simulink subsystem "rss_RefTqLimCalc"  (R2023a)
settings: Solver=VariableStepAuto  StartTime=0.0  StopTime=inf  RelTol=1e-3
undefined symbols (not defined in the file): bit, Cdbl_iPhCurrMaxVal, Cdbl_iPhCurrPeakVal, Cdbl_iSplyCurrMaxVal, Cdbl_numPPNumMaxVal, Cdbl_psiPermMagFlxMaxVal, Cdbl_psiPermMagFlxMinVal, Cdbl_psiPermMagFlxPeakVal, Cdbl_trqTqMaxVal, Cdbl_trqTqPeakVal, Cdbl_uPhVltgMaxVal, Cdbl_uSplyVltgMaxVal, Gs16_iPhCurrLim_CUR, Gs16_iPhCurrLim_CUR_tPCBTemp_X, Gs16_iSplyCurrTempLim_CUR, Gs16_iSplyCurrTempLim_CUR_tPCBTemp_X, Gs16_iSplyCurrVltgLim_CUR, Gs16_iSplyCurrVltgLim_CUR_uSplyVltg_X
libraries: lib_conversion x9, lib_configurable_parameter x3, lib_dynamic_saturator x2, simulink x1, lib_iir_filter x1
settings Model: DefaultTestHarness=rss_DeratingControl_thu  Creator=CAV2OFO  LastModifiedBy=xiaoqiang.yuan
settings OptimizationCC: ReuseModelBlockBuffer=off

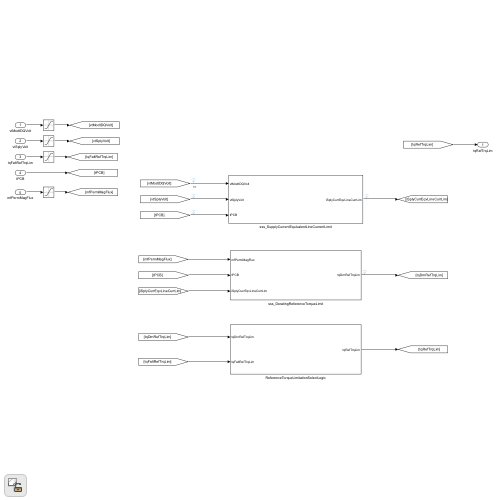
[thumbnail: Simulink's stored preview of the top-level diagram]
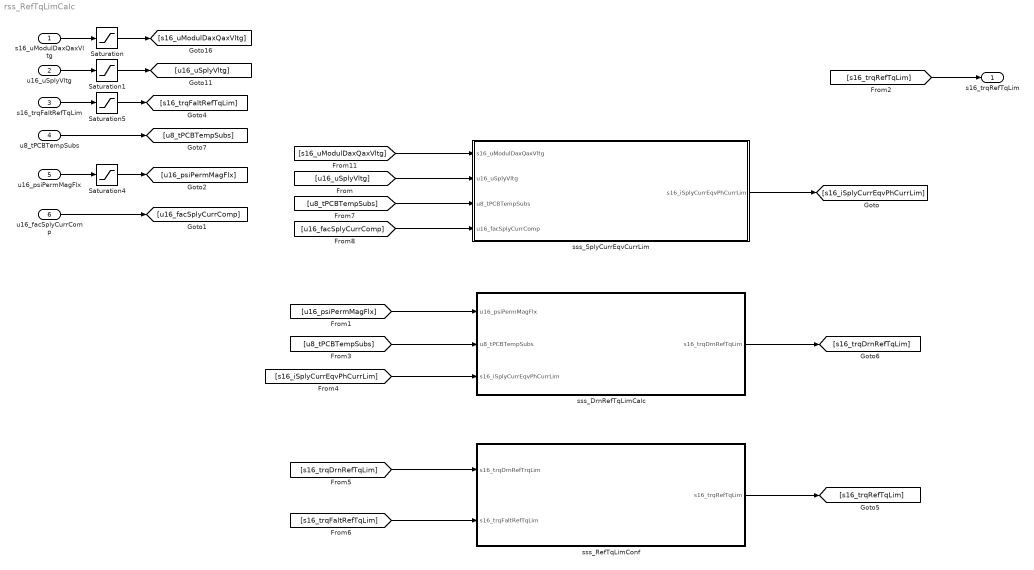
== system rss_RefTqLimCalc ==
  s16_uModulDaxQaxVltg : Inport  OutDataTypeStr=dt_Standardize_s16p15b0
  u16_uSplyVltg : Inport  Port=2  OutDataTypeStr=dt_Standardize_u16p15b0
  s16_trqFaltRefTqLim : Inport  Port=3  OutDataTypeStr=dt_Standardize_s16p15b0
  u8_tPCBTempSubs : Inport  Port=4  OutDataTypeStr=dt_Temp_u8p0bn40
  u16_psiPermMagFlx : Inport  Port=5  OutDataTypeStr=dt_Standardize_u16p15b0
  u16_facSplyCurrComp : Inport  Port=6  OutDataTypeStr=dt_Standardize_u16p15b0
  Saturation : Saturate  UpperLimit=Cdbl_uPhVltgMaxVal  LowerLimit=-Cdbl_uPhVltgMaxVal
  Saturation1 : Saturate  UpperLimit=Cdbl_uSplyVltgMaxVal  LowerLimit=0
  Saturation4 : Saturate  UpperLimit=Cdbl_psiPermMagFlxMaxVal  LowerLimit=Cdbl_psiPermMagFlxMinVal
  Saturation5 : Saturate  UpperLimit=Cdbl_trqTqMaxVal  LowerLimit=-Cdbl_trqTqMaxVal  LinearizeAsGain=off
  sss_DrnRefTqLimCalc : Subsystem
  sss_RefTqLimConf : Subsystem
  sss_SplyCurrEqvCurrLim : Subsystem
  s16_trqRefTqLim : Outport  OutDataTypeStr=dt_Standardize_s16p15b0
  wires:
  [s16_trqRefTqLim] -> s16_trqRefTqLim/1
  s16_uModulDaxQaxVltg/1 -> Saturation/1
  u16_uSplyVltg/1 -> Saturation1/1
  [u16_uSplyVltg] -> sss_SplyCurrEqvCurrLim/2(u16_uSplyVltg)
  [s16_uModulDaxQaxVltg] -> sss_SplyCurrEqvCurrLim/1(s16_uModulDaxQaxVltg)
  sss_SplyCurrEqvCurrLim/1(s16_iSplyCurrEqvPhCurrLim) -> [s16_iSplyCurrEqvPhCurrLim]
  [u16_psiPermMagFlx] -> sss_DrnRefTqLimCalc/1(u16_psiPermMagFlx)
  [u8_tPCBTempSubs] -> sss_DrnRefTqLimCalc/2(u8_tPCBTempSubs)
  [s16_iSplyCurrEqvPhCurrLim] -> sss_DrnRefTqLimCalc/3(s16_iSplyCurrEqvPhCurrLim)
  Saturation/1 -> [s16_uModulDaxQaxVltg]
  Saturation1/1 -> [u16_uSplyVltg]
  Saturation4/1 -> [u16_psiPermMagFlx]
  s16_trqFaltRefTqLim/1 -> Saturation5/1
  Saturation5/1 -> [s16_trqFaltRefTqLim]
  sss_RefTqLimConf/1(s16_trqRefTqLim) -> [s16_trqRefTqLim]
  sss_DrnRefTqLimCalc/1(s16_trqDrnRefTqLim) -> [s16_trqDrnRefTqLim]
  [s16_trqDrnRefTqLim] -> sss_RefTqLimConf/1(s16_trqDrnRefTrqLim)
  [s16_trqFaltRefTqLim] -> sss_RefTqLimConf/2(s16_trqFaltRefTqLim)
  u8_tPCBTempSubs/1 -> [u8_tPCBTempSubs]
  [u8_tPCBTempSubs] -> sss_SplyCurrEqvCurrLim/3(u8_tPCBTempSubs)
  u16_psiPermMagFlx/1 -> Saturation4/1
  u16_facSplyCurrComp/1 -> [u16_facSplyCurrComp]
  [u16_facSplyCurrComp] -> sss_SplyCurrEqvCurrLim/4(u16_facSplyCurrComp)

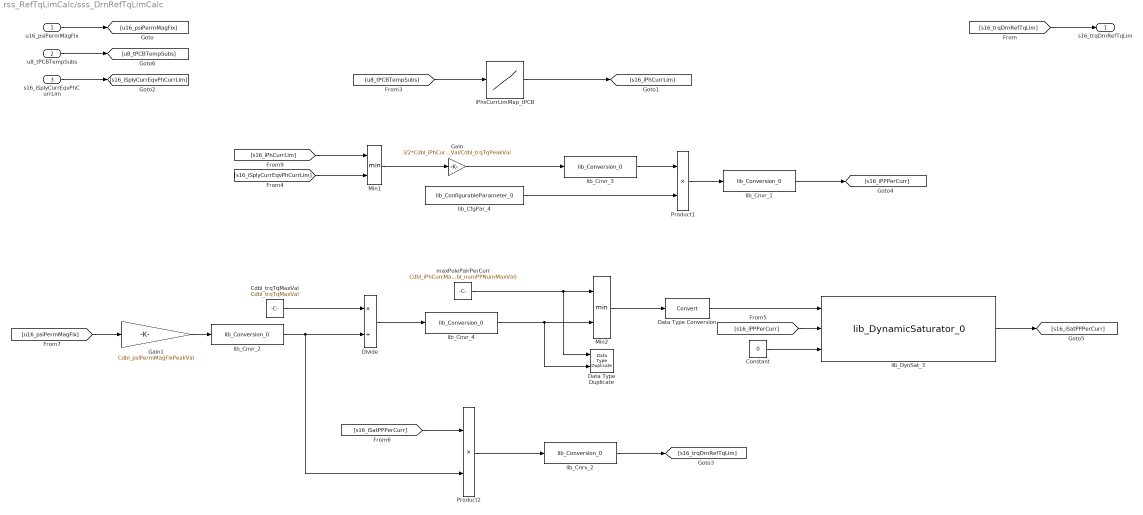
== system rss_RefTqLimCalc/sss_DrnRefTqLimCalc ==
  u16_psiPermMagFlx : Inport
  u8_tPCBTempSubs : Inport  Port=2
  s16_iSplyCurrEqvPhCurrLim : Inport  Port=3
  Cdbl_trqTqMaxVal : Constant  Value=Cdbl_trqTqMaxVal  OutDataTypeStr=dt_Standardize_s16p15b0
  Constant : Constant  Value=0  OutDataTypeStr=Inherit: Inherit via back propagation
  Data Type Duplicate : DataTypeDuplicate
  Data Type Conversion : DataTypeConversion  SaturateOnIntegerOverflow=off  RndMeth=Floor
  Divide : Product  Inputs=*/  OutDataTypeStr=Inherit: Inherit via back propagation  RndMeth=Simplest
  Gain : Gain  Gain=3/2*Cdbl_iPhCurrPeakVal/Cdbl_trqTqPeakVal  OutDataTypeStr=Inherit: Inherit via back propagation
  Gain1 : Gain  Gain=Cdbl_psiPermMagFlxPeakVal  OutDataTypeStr=Inherit: Inherit via back propagation
  Min1 : MinMax  Inputs=2
  Min2 : MinMax  Inputs=2
  Product1 : Product  OutDataTypeStr=Inherit: Inherit via back propagation
  Product2 : Product  OutDataTypeStr=dt_Standardize_s16p15b0
  iPhsCurrLimMap_tPCB : Lookup_n-D  NumberOfTableDimensions=1  BreakpointsForDimension1=Gs16_iPhCurrLim_CUR_tPCBTemp_X  Table=Gs16_iPhCurrLim_CUR  ExtrapMethod=Clip  InternalRulePriority=Speed  OutDataTypeStr=Inherit: Inherit from 'Table data'  RndMeth=Simplest
  lib_CfgPar_4 : lib_configurable_parameter/lib_ConfigurableParameter_0  lb_parCnfgPar=Gu8_numPPNum_C  lb_parDataType=Inherit: Inherit from 'Constant value'  lb_parUpLim=Cdbl_numPPNumMaxVal  lb_parLowLim=Cdbl_numPPNumMinVal
  lib_Cnrv_2 : lib_conversion/lib_Conversion_0  lb_parDataType=dt_Standardize_s16p15b0  lb_parOutpMaxVal=[]  lb_parOutpMinVal=[]  RndMeth=Simplest  lb_parSatFlag=off
  lib_Cnvr_1 : lib_conversion/lib_Conversion_0  lb_parDataType=fixdt(0,16)  lb_parOutpMaxVal=Cdbl_iPhCurrMaxVal*3/2*Cdbl_iPhCurrPeakVal/Cdbl_trqTqPeakVal*double(Cdbl_numPPNumMaxVal)  lb_parOutpMinVal=[]  RndMeth=Simplest  lb_parSatFlag=off
  lib_Cnvr_2 : lib_conversion/lib_Conversion_0  lb_parDataType=fixdt(0,16)  lb_parOutpMaxVal=Cdbl_psiPermMagFlxPeakVal  lb_parOutpMinVal=[]  RndMeth=Simplest  lb_parSatFlag=off
  lib_Cnvr_3 : lib_conversion/lib_Conversion_0  lb_parDataType=fixdt(0,16)  lb_parOutpMaxVal=Cdbl_iPhCurrMaxVal*3/2*Cdbl_iPhCurrPeakVal/Cdbl_trqTqPeakVal  lb_parOutpMinVal=[]  RndMeth=Simplest  lb_parSatFlag=off
  lib_Cnvr_4 : lib_conversion/lib_Conversion_0  lb_parDataType=fixdt(0,16)  lb_parOutpMaxVal=Cdbl_trqTqMaxVal/Cdbl_psiPermMagFlxMinVal  lb_parOutpMinVal=[]  RndMeth=Simplest  lb_parSatFlag=off
  lib_DynSat_3 : lib_dynamic_saturator/lib_DynamicSaturator_0
  maxPolePairPerCurr : Constant  Value=Cdbl_iPhCurrMaxVal*3/2*Cdbl_iPhCurrPeakVal/Cdbl_trqTqPeakVal*double(Cdbl_numPPNumMaxVal)  OutDataTypeStr=Inherit: Inherit via back propagation
  s16_trqDrnRefTqLim : Outport
  wires:
  [u16_psiPermMagFlx] -> Gain1/1
  Gain1/1 -> lib_Cnvr_2/1
  iPhsCurrLimMap_tPCB/1 -> [s16_iPhCurrLim]
  [u8_tPCBTempSubs] -> iPhsCurrLimMap_tPCB/1
  u8_tPCBTempSubs/1 -> [u8_tPCBTempSubs]
  lib_Cnrv_2/1 -> [s16_trqDrnRefTqLim]
  Min2/1 -> Data Type Conversion/1
  maxPolePairPerCurr/1 -> Min2/1, Data Type Duplicate/1
  Data Type Conversion/1 -> lib_DynSat_3/1
  lib_Cnvr_4/1 -> Min2/2, Data Type Duplicate/2
  lib_Cnvr_3/1 -> Product1/1
  [s16_iSatPPPerCurr] -> Product2/1
  lib_DynSat_3/1 -> [s16_iSatPPPerCurr]
  [s16_iPPPerCurr] -> lib_DynSat_3/2
  Divide/1 -> lib_Cnvr_4/1
  lib_Cnvr_1/1 -> [s16_iPPPerCurr]
  Cdbl_trqTqMaxVal/1 -> Divide/1
  Constant/1 -> lib_DynSat_3/3
  [s16_trqDrnRefTqLim] -> s16_trqDrnRefTqLim/1
  s16_iSplyCurrEqvPhCurrLim/1 -> [s16_iSplyCurrEqvPhCurrLim]
  [s16_iSplyCurrEqvPhCurrLim] -> Min1/2
  [s16_iPhCurrLim] -> Min1/1
  u16_psiPermMagFlx/1 -> [u16_psiPermMagFlx]
  Product2/1 -> lib_Cnrv_2/1
  Product1/1 -> lib_Cnvr_1/1
  Gain/1 -> lib_Cnvr_3/1
  lib_CfgPar_4/1 -> Product1/2
  Min1/1 -> Gain/1
  lib_Cnvr_2/1 -> Product2/2, Divide/2

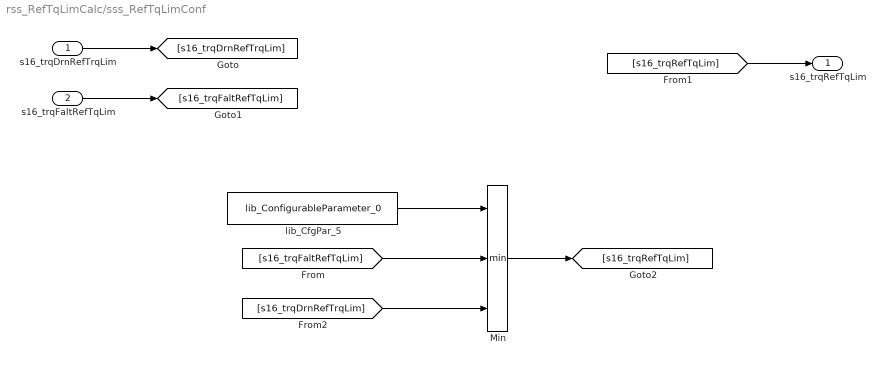
== system rss_RefTqLimCalc/sss_RefTqLimConf ==
  s16_trqDrnRefTrqLim : Inport
  s16_trqFaltRefTqLim : Inport  Port=2
  Min : MinMax  Inputs=3
  lib_CfgPar_5 : lib_configurable_parameter/lib_ConfigurableParameter_0  lb_parCnfgPar=Gs16_trqTqUpLim_C  lb_parDataType=Inherit: Inherit from 'Constant value'  lb_parUpLim=Cdbl_trqTqMaxVal  lb_parLowLim=0
  s16_trqRefTqLim : Outport
  wires:
  Min/1 -> [s16_trqRefTqLim]
  [s16_trqRefTqLim] -> s16_trqRefTqLim/1
  [s16_trqDrnRefTrqLim] -> Min/3
  s16_trqFaltRefTqLim/1 -> [s16_trqFaltRefTqLim]
  [s16_trqFaltRefTqLim] -> Min/2
  s16_trqDrnRefTrqLim/1 -> [s16_trqDrnRefTrqLim]
  lib_CfgPar_5/1 -> Min/1

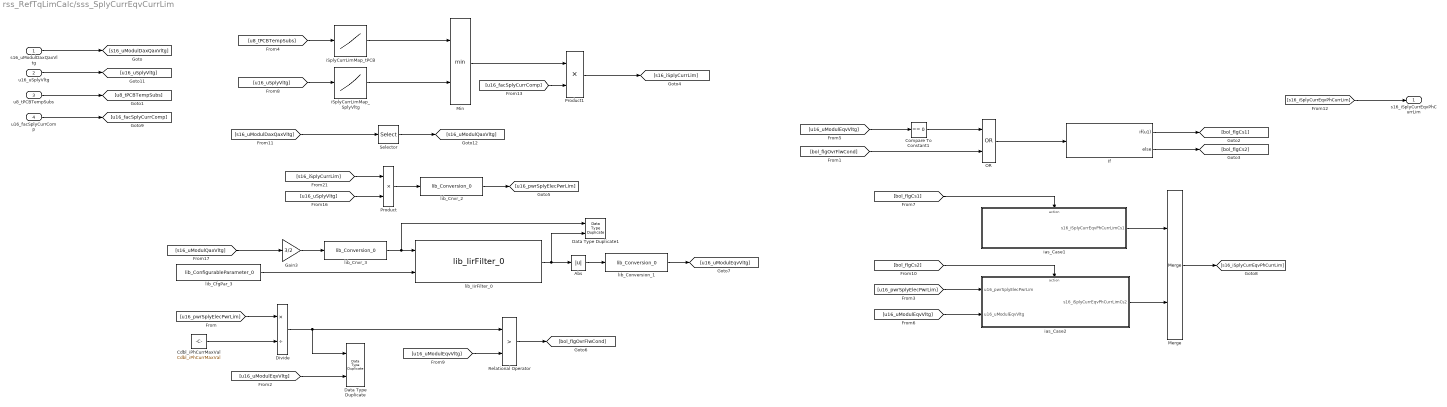
== system rss_RefTqLimCalc/sss_SplyCurrEqvCurrLim ==
  s16_uModulDaxQaxVltg : Inport
  u16_uSplyVltg : Inport  Port=2
  u8_tPCBTempSubs : Inport  Port=3
  u16_facSplyCurrComp : Inport  Port=4
  Abs : Abs  OutDataTypeStr=Inherit: Inherit via back propagation  RndMeth=Simplest  SaturateOnIntegerOverflow=off
  Cdbl_iPhCurrMaxVal : Constant  Value=Cdbl_iPhCurrMaxVal  OutDataTypeStr=dt_Standardize_s16p15b0
  Compare To Constant1 : simulink/Logic and Bit Operations/Compare To Constant  relop===  const=0  OutDataTypeStr=boolean
  Data Type Duplicate : DataTypeDuplicate
  Data Type Duplicate1 : DataTypeDuplicate
  Divide : Product  Inputs=*/  OutDataTypeStr=Inherit: Inherit via back propagation  RndMeth=Simplest
  Gain3 : Gain  Gain=3/2  OutDataTypeStr=Inherit: Inherit via back propagation  RndMeth=Simplest
  If : If  IfExpression=u1
  Merge : Merge
  Min : MinMax  Inputs=2
  OR : Logic  Operator=OR  AllPortsSameDT=off  OutDataTypeStr=boolean
  Product : Product  OutDataTypeStr=Inherit: Inherit via back propagation  RndMeth=Simplest
  Product1 : Product  RndMeth=Simplest  OutDataTypeStr=Inherit: Same as first input
  Relational Operator : RelationalOperator  Operator=>  OutDataTypeStr=boolean  RndMeth=Simplest  InputSameDT=off
  Selector : Selector  IndexMode=Zero-based  InputPortWidth=2  IndexOptions=Index vector (dialog)  Indices=1  OutputSizes=1
  iSplyCurrLimMap_SplyVltg : Lookup_n-D  NumberOfTableDimensions=1  BreakpointsForDimension1=Gs16_iSplyCurrVltgLim_CUR_uSplyVltg_X  Table=Gs16_iSplyCurrVltgLim_CUR  ExtrapMethod=Clip  InternalRulePriority=Speed  OutDataTypeStr=Inherit: Inherit from 'Table data'  RndMeth=Simplest
  iSplyCurrLimMap_tPCB : Lookup_n-D  NumberOfTableDimensions=1  BreakpointsForDimension1=Gs16_iSplyCurrTempLim_CUR_tPCBTemp_X  Table=Gs16_iSplyCurrTempLim_CUR  ExtrapMethod=Clip  InternalRulePriority=Speed  OutDataTypeStr=Inherit: Inherit from 'Table data'  RndMeth=Simplest
  ias_Case1 : Subsystem  TreatAsAtomicUnit=on
  ias_Case2 : Subsystem  TreatAsAtomicUnit=on
  lib_CfgPar_3 : lib_configurable_parameter/lib_ConfigurableParameter_0  lb_parCnfgPar=Gu16_facDrtnVltgFltCoeff_C  lb_parDataType=Inherit: Inherit from 'Constant value'  lb_parUpLim=Cdbl_facDrtnVltgFltCoeffMaxVal  lb_parLowLim=0
  lib_Cnvr_2 : lib_conversion/lib_Conversion_0  lb_parDataType=fixdt(0,16)  lb_parOutpMaxVal=Cdbl_iSplyCurrMaxVal*Cdbl_uSplyVltgMaxVal  lb_parOutpMinVal=[]  lb_parSatFlag=off
  lib_Cnvr_3 : lib_conversion/lib_Conversion_0  lb_parDataType=fixdt(1,16)  lb_parOutpMaxVal=3/2*Cdbl_uPhVltgMaxVal  lb_parOutpMinVal=[]  lb_parSatFlag=off
  lib_Conversion_1 : lib_conversion/lib_Conversion_0  lb_parDataType=fixdt(0,16)  lb_parOutpMaxVal=3/2*Cdbl_uPhVltgMaxVal  lb_parOutpMinVal=[]  lb_parSatFlag=off
  lib_IirFilter_0 : lib_iir_filter/lib_IirFilter_0  lb_parMaxInpVal=3/2*Cdbl_uPhVltgMaxVal  lb_parFltrCoefMaxVal=Cdbl_facDrtnVltgFltCoeffMaxVal  lb_parBitNumMode=32-bit  lb_parOutpDataType=Inherit: Inherit via back propagation  lb_parFiltTypeMode=Low-pass
  s16_iSplyCurrEqvPhCurrLim : Outport
  wires:
  Product1/1 -> [s16_iSplyCurrLim]
  Min/1 -> Product1/1
  [u16_facSplyCurrComp] -> Product1/2
  u16_facSplyCurrComp/1 -> [u16_facSplyCurrComp]
  [s16_iSplyCurrEqvPhCurrLim] -> s16_iSplyCurrEqvPhCurrLim/1
  Merge/1 -> [s16_iSplyCurrEqvPhCurrLim]
  iSplyCurrLimMap_SplyVltg/1 -> Min/2
  iSplyCurrLimMap_tPCB/1 -> Min/1
  [u16_uSplyVltg] -> iSplyCurrLimMap_SplyVltg/1
  [u8_tPCBTempSubs] -> iSplyCurrLimMap_tPCB/1
  u8_tPCBTempSubs/1 -> [u8_tPCBTempSubs]
  [u16_uModulEqvVltg] -> Data Type Duplicate/2
  lib_Cnvr_3/1 -> Data Type Duplicate1/1, lib_IirFilter_0/1
  u16_uSplyVltg/1 -> [u16_uSplyVltg]
  s16_uModulDaxQaxVltg/1 -> [s16_uModulDaxQaxVltg]
  lib_Cnvr_2/1 -> [u16_pwrSplyElecPwrLim]
  Divide/1 -> Relational Operator/1, Data Type Duplicate/1
  [bol_flgOvrFlwCond] -> OR/2
  Relational Operator/1 -> [bol_flgOvrFlwCond]
  Compare To Constant1/1 -> OR/1
  [u16_uModulEqvVltg] -> Relational Operator/2
  [u16_uModulEqvVltg] -> ias_Case2/2(u16_uModulEqvVltg)
  [u16_pwrSplyElecPwrLim] -> ias_Case2/1(u16_pwrSplyElecPwrLim)
  [u16_pwrSplyElecPwrLim] -> Divide/1
  Product/1 -> lib_Cnvr_2/1
  [s16_uModulQaxVltg] -> Gain3/1
  Gain3/1 -> lib_Cnvr_3/1
  lib_CfgPar_3/1 -> lib_IirFilter_0/2
  Cdbl_iPhCurrMaxVal/1 -> Divide/2
  [s16_iSplyCurrLim] -> Product/1
  [u16_uSplyVltg] -> Product/2
  ias_Case2/1(s16_iSplyCurrEqvPhCurrLimCs2) -> Merge/2
  ias_Case1/1(s16_iSplyCurrEqvPhCurrLimCs1) -> Merge/1
  [bol_flgCs2] -> ias_Case2/Action
  If/2 -> [bol_flgCs2]
  [bol_flgCs1] -> ias_Case1/Action
  If/1 -> [bol_flgCs1]
  OR/1 -> If/1
  [u16_uModulEqvVltg] -> Compare To Constant1/1
  [s16_uModulDaxQaxVltg] -> Selector/1
  Selector/1 -> [s16_uModulQaxVltg]
  lib_IirFilter_0/1 -> Abs/1, Data Type Duplicate1/2
  Abs/1 -> lib_Conversion_1/1
  lib_Conversion_1/1 -> [u16_uModulEqvVltg]

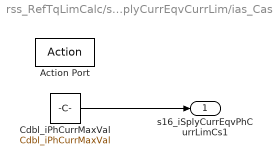
== system rss_RefTqLimCalc/sss_SplyCurrEqvCurrLim/ias_Case1 ==
  Action Port : ActionPort
  Cdbl_iPhCurrMaxVal : Constant  Value=Cdbl_iPhCurrMaxVal  OutDataTypeStr=dt_Standardize_s16p15b0
  s16_iSplyCurrEqvPhCurrLimCs1 : Outport
  wires:
  Cdbl_iPhCurrMaxVal/1 -> s16_iSplyCurrEqvPhCurrLimCs1/1

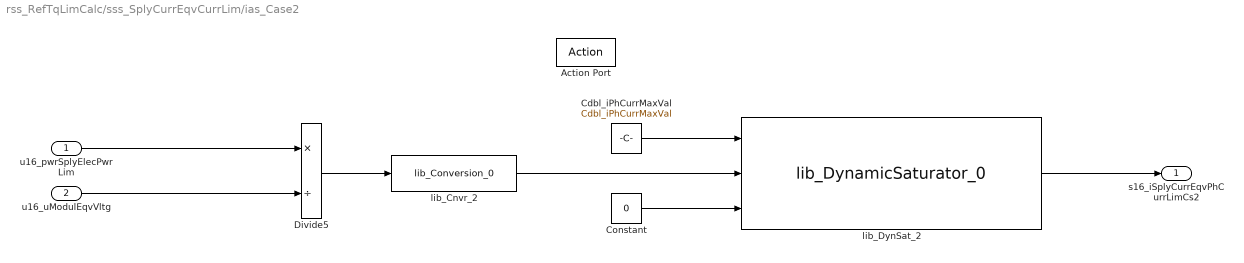
== system rss_RefTqLimCalc/sss_SplyCurrEqvCurrLim/ias_Case2 ==
  u16_pwrSplyElecPwrLim : Inport
  u16_uModulEqvVltg : Inport  Port=2
  Action Port : ActionPort
  Cdbl_iPhCurrMaxVal : Constant  Value=Cdbl_iPhCurrMaxVal  OutDataTypeStr=dt_Standardize_s16p15b0
  Constant : Constant  Value=0  OutDataTypeStr=dt_Standardize_s16p15b0
  Divide5 : Product  Inputs=*/  OutDataTypeStr=Inherit: Inherit via back propagation  RndMeth=Simplest
  lib_Cnvr_2 : lib_conversion/lib_Conversion_0  lb_parDataType=Inherit: Inherit via back propagation  lb_parOutpMaxVal=[]  lb_parOutpMinVal=[]  RndMeth=Simplest  lb_parSatFlag=off
  lib_DynSat_2 : lib_dynamic_saturator/lib_DynamicSaturator_0
  s16_iSplyCurrEqvPhCurrLimCs2 : Outport
  wires:
  lib_Cnvr_2/1 -> lib_DynSat_2/2
  lib_DynSat_2/1 -> s16_iSplyCurrEqvPhCurrLimCs2/1
  Cdbl_iPhCurrMaxVal/1 -> lib_DynSat_2/1
  Constant/1 -> lib_DynSat_2/3
  Divide5/1 -> lib_Cnvr_2/1
  u16_pwrSplyElecPwrLim/1 -> Divide5/1
  u16_uModulEqvVltg/1 -> Divide5/2
